simulink model "GS_Flare"  (R2022a)
settings: Solver=VariableStepAuto  StartTime=0.0  StopTime=180  RelTol=1e-3
values from neighbouring files (symbols this model uses):
  A_long = SS_lo.A([3 7 8 5 11], [3 7 8 5 11])    [glideslope_flare.m]    (also in openloop_pitchrate.m = SS_lo.A([7 8 5 11], [7 8 5 11]))
  B_long = SS_lo.A([3 7 8 5 11], [13, 14])    [glideslope_flare.m]    (also in openloop_pitchrate.m = SS_lo.A([7 8 5 11], 14))
  C_long = SS_lo.C([3 7 8 5 11], [3 7 8 5 11])    [glideslope_flare.m]    (also in openloop_pitchrate.m = SS_lo.C([7 8 5 11], [7 8 5 11]))
  D_long = SS_lo.C([3 7 8 5 11], [13, 14])    [glideslope_flare.m]    (also in openloop_pitchrate.m = SS_lo.C([7 8 5 11], 14))
  ho = 9.44    [glideslope_flare.m]
  tau = 3.15    [glideslope_flare.m]
undefined symbols (not defined in the file or in its folder): magnitude
libraries: simulink_extras x3, slpidlib x1
settings Model: Creator=gabri  LastModifiedBy=gabri

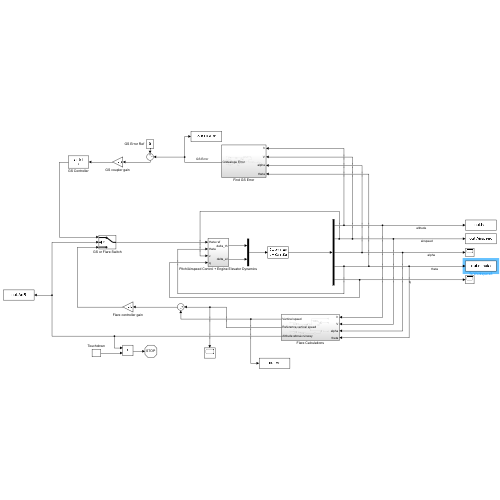
[thumbnail: Simulink's stored preview of the top-level diagram]
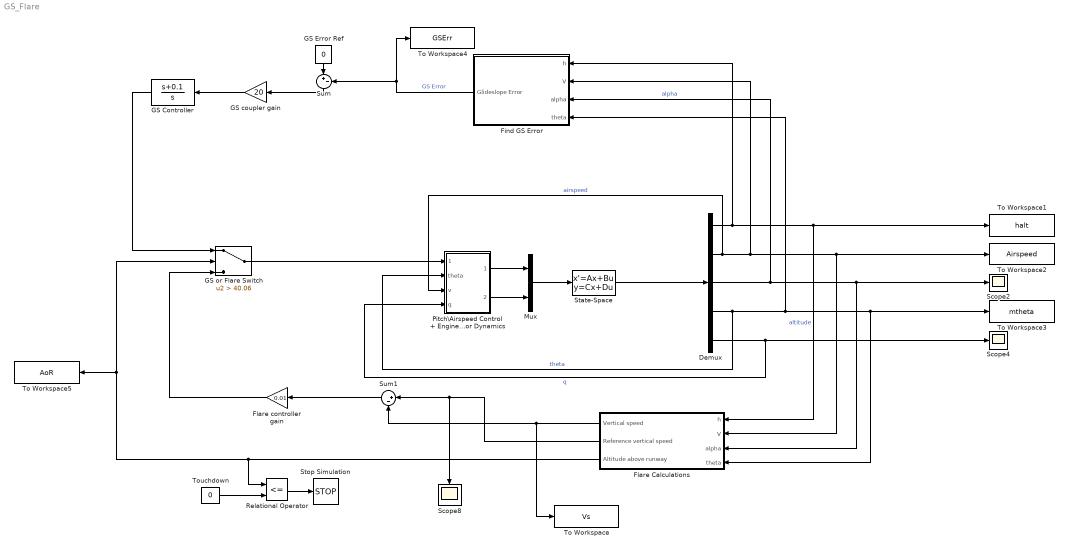
== system GS_Flare ==
  Demux : Demux  Outputs=5
  Find GS Error : Subsystem
  Flare Calculations : Subsystem
  Flare controller gain : Gain  Gain=0.01
  GS Controller : TransferFcn  Numerator=[1 0.1]  Denominator=[1 0]
  GS Error Ref : Constant  Value=0
  GS coupler gain : Gain  Gain=20
  GS or Flare Switch : Switch  Criteria=u2 > Threshold  Threshold=40.06  SaturateOnIntegerOverflow=off  InputSameDT=off
  Mux : Mux  Inputs=2
  Pitch\Airspeed Control + Engine Elevator Dynamics : Subsystem
  Relational Operator : RelationalOperator  Operator=<=  OutDataTypeStr=boolean  RndMeth=Simplest  InputSameDT=off
  Scope2 : Scope
  Scope4 : Scope
  Scope8 : Scope
  State-Space : StateSpace  A=A_long  B=B_long  C=C_long  D=D_long  InitialCondition=0
  Stop Simulation : Stop
  Sum : Sum  Inputs=|+-
  Sum1 : Sum  Inputs=|+-
  To Workspace : ToWorkspace  VariableName=Vs  SaveFormat=Timeseries  SampleTime=-1
  To Workspace1 : ToWorkspace  VariableName=halt  SaveFormat=Timeseries  SampleTime=-1
  To Workspace2 : ToWorkspace  VariableName=Airspeed  SaveFormat=Timeseries  SampleTime=-1
  To Workspace3 : ToWorkspace  VariableName=mtheta  SaveFormat=Timeseries  SampleTime=-1
  To Workspace4 : ToWorkspace  VariableName=GSErr  SaveFormat=Timeseries  SampleTime=-1
  To Workspace5 : ToWorkspace  VariableName=AoR  SaveFormat=Timeseries  SampleTime=-1
  Touchdown : Constant  Value=0
  wires:
  Demux/1 -> To Workspace1/1, Flare Calculations/1(h), Find GS Error/1(h)  "altitude"
  Demux/5 -> Pitch\Airspeed Control + Engine Elevator Dynamics/4(q), Scope4/1  "q"
  Demux/4 -> Pitch\Airspeed Control + Engine Elevator Dynamics/2(theta), To Workspace3/1, Flare Calculations/4(theta), Find GS Error/4(theta)  "theta"
  Demux/3 -> Flare Calculations/3(alpha), Scope2/1, Find GS Error/3(alpha)  "alpha"
  Demux/2 -> To Workspace2/1, Flare Calculations/2(V), Find GS Error/2(V), Pitch\Airspeed Control + Engine Elevator Dynamics/3(v)  "airspeed"
  State-Space/1 -> Demux/1
  Mux/1 -> State-Space/1
  Pitch\Airspeed Control + Engine Elevator Dynamics/2(delta_el) -> Mux/2
  Find GS Error/1(Glideslope Error) -> To Workspace4/1, Sum/2  "GS Error"
  GS Controller/1 -> GS or Flare Switch/1
  Sum/1 -> GS coupler gain/1
  GS coupler gain/1 -> GS Controller/1
  Flare Calculations/3(Altitude above runway) -> Relational Operator/1, To Workspace5/1, GS or Flare Switch/2
  Flare Calculations/2(Reference vertical speed) -> Sum1/1, Scope8/1
  Flare Calculations/1(Vertical speed) -> To Workspace/1, Sum1/2
  GS or Flare Switch/1 -> Pitch\Airspeed Control + Engine Elevator Dynamics/1(theta ref)
  GS Error Ref/1 -> Sum/1
  Relational Operator/1 -> Stop Simulation/1
  Touchdown/1 -> Relational Operator/2
  Sum1/1 -> Flare controller gain/1
  Flare controller gain/1 -> GS or Flare Switch/3
  Pitch\Airspeed Control + Engine Elevator Dynamics/1(delta_th) -> Mux/1

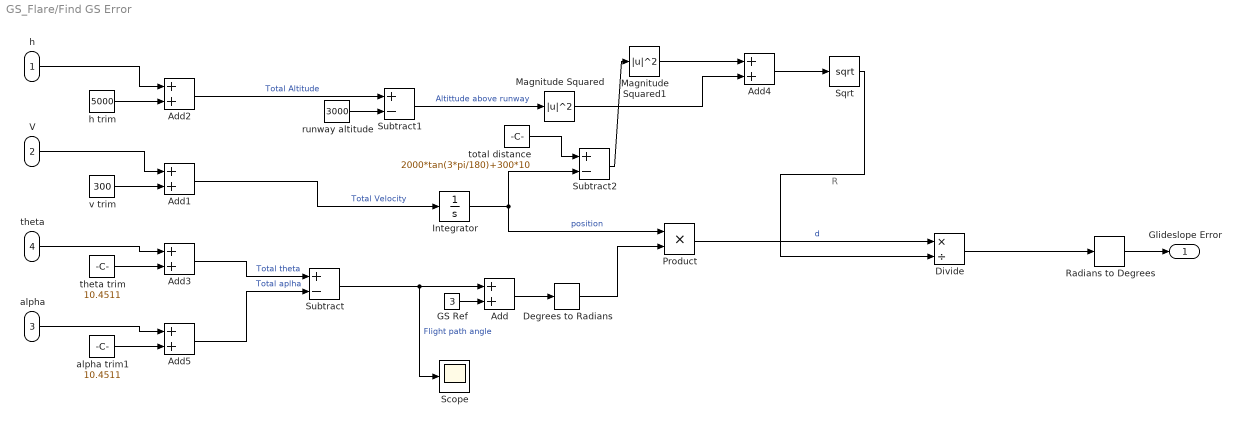
== system GS_Flare/Find GS Error ==
  note: R
  h : Inport
  V : Inport  Port=2
  alpha : Inport  Port=3
  theta : Inport  Port=4
  Add{,1..5} (6 alike) : Sum
  Degrees to Radians : simulink_extras/Transformations/Degrees to Radians
  Divide : Product  Inputs=*/
  GS Ref : Constant  Value=3
  Integrator : Integrator
  Magnitude Squared : Math  Operator=magnitude^2
  Magnitude Squared1 : Math  Operator=magnitude^2
  Product : Product
  Radians to Degrees : simulink_extras/Transformations/Radians to Degrees
  Scope : Scope
  Sqrt : Sqrt
  Subtract : Sum  Inputs=+-
  Subtract1 : Sum  Inputs=+-
  Subtract2 : Sum  Inputs=+-
  alpha trim1 : Constant  Value=10.4511
  h trim : Constant  Value=5000
  runway altitude : Constant  Value=3000
  theta trim : Constant  Value=10.4511
  total distance : Constant  Value=2000*tan(3*pi/180)+300*10
  v trim : Constant  Value=300
  Glideslope Error : Outport
  wires:
  h trim/1 -> Add2/2
  Add1/1 -> Integrator/1  "Total Velocity"
  theta/1 -> Add3/1
  V/1 -> Add1/1
  alpha trim1/1 -> Add5/2
  Product/1 -> Divide/1  "d"
  v trim/1 -> Add1/2
  Add2/1 -> Subtract1/1  "Total Altitude"
  h/1 -> Add2/1
  Radians to Degrees/1 -> Glideslope Error/1
  Subtract/1 -> Scope/1, Add/1  "Flight path angle"
  Add3/1 -> Subtract/1  "Total theta"
  Add/1 -> Degrees to Radians/1
  Degrees to Radians/1 -> Product/2
  Divide/1 -> Radians to Degrees/1
  alpha/1 -> Add5/1
  theta trim/1 -> Add3/2
  GS Ref/1 -> Add/2
  Add5/1 -> Subtract/2  "Total aplha"
  Subtract1/1 -> Magnitude Squared/1  "Altittude above runway"
  Magnitude Squared1/1 -> Add4/1
  Add4/1 -> Sqrt/1
  runway altitude/1 -> Subtract1/2
  Magnitude Squared/1 -> Add4/2
  Sqrt/1 -> Divide/2
  Integrator/1 -> Product/1, Subtract2/2  "position"
  Subtract2/1 -> Magnitude Squared1/1
  total distance/1 -> Subtract2/1

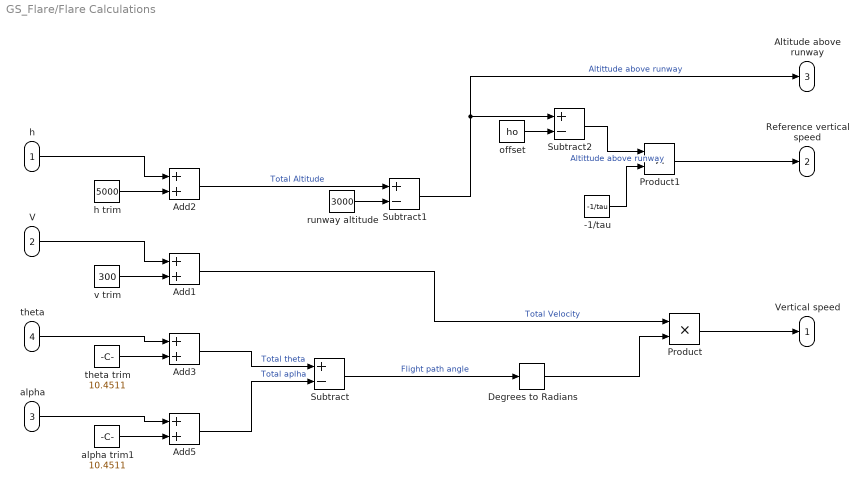
== system GS_Flare/Flare Calculations ==
  h : Inport
  V : Inport  Port=2
  alpha : Inport  Port=3
  theta : Inport  Port=4
  -1/tau : Constant  Value=-1/tau
  Add{1..3,5} (4 alike) : Sum
  Degrees to Radians : simulink_extras/Transformations/Degrees to Radians
  Product : Product
  Product1 : Product
  Subtract : Sum  Inputs=+-
  Subtract1 : Sum  Inputs=+-
  Subtract2 : Sum  Inputs=+-
  alpha trim1 : Constant  Value=10.4511
  h trim : Constant  Value=5000
  offset : Constant  Value=ho
  runway altitude : Constant  Value=3000
  theta trim : Constant  Value=10.4511
  v trim : Constant  Value=300
  Vertical speed : Outport
  Reference vertical speed : Outport  Port=2
  Altitude above runway : Outport  Port=3
  wires:
  alpha trim1/1 -> Add5/2
  -1/tau/1 -> Product1/2
  Degrees to Radians/1 -> Product/2
  Product1/1 -> Reference vertical speed/1
  theta/1 -> Add3/1
  runway altitude/1 -> Subtract1/2
  Add5/1 -> Subtract/2  "Total aplha"
  h trim/1 -> Add2/2
  alpha/1 -> Add5/1
  Subtract1/1 -> Subtract2/1, Altitude above runway/1  "Altittude above runway"
  v trim/1 -> Add1/2
  theta trim/1 -> Add3/2
  V/1 -> Add1/1
  h/1 -> Add2/1
  Add3/1 -> Subtract/1  "Total theta"
  Add2/1 -> Subtract1/1  "Total Altitude"
  Product/1 -> Vertical speed/1
  Subtract/1 -> Degrees to Radians/1  "Flight path angle"
  Add1/1 -> Product/1  "Total Velocity"
  Subtract2/1 -> Product1/1  "Altittude above runway"
  offset/1 -> Subtract2/2

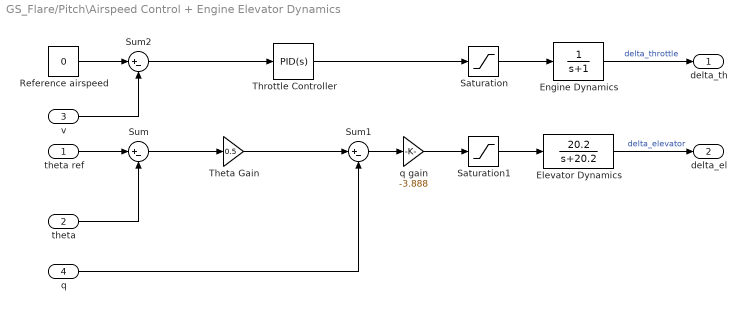
== system GS_Flare/Pitch\Airspeed Control + Engine Elevator Dynamics ==
  theta ref : Inport
  theta : Inport  Port=2
  v : Inport  Port=3
  q : Inport  Port=4
  Elevator Dynamics : TransferFcn  Numerator=[20.2]  Denominator=[1 20.2]
  Engine Dynamics : TransferFcn  Denominator=[1 1]
  Reference airspeed : Constant  Value=0
  Saturation : Saturate  UpperLimit=19000-2826.8165  LowerLimit=1000-2826.8165
  Saturation1 : Saturate  UpperLimit=25+4.1891  LowerLimit=-25+4.1891
  Sum : Sum  Inputs=|+-
  Sum1 : Sum  Inputs=|+-
  Sum2 : Sum  Inputs=|+-
  Theta Gain : Gain  Gain=0.5
  Throttle Controller : slpidlib/PID Controller  Controller=PID  Form=Parallel  TimeDomain=Continuous-time  UseExternalTs=off  SampleTime=-1  IntegratorMethod=Forward Euler  FilterMethod=Forward Euler  ControllerParametersSource=internal  P=5000  I=20  UseKiTs=off  D=100  N=100  UseFilter=on  TunerSelectOption=Transfer Function Based (PID Tuner App)  InitialConditionSource=internal  InitialConditionForIntegrator=0  InitialConditionForFilter=0  DifferentiatorICPrevScaledInput=0  ExternalReset=none  TrackingMode=off  Kt=1  LimitOutput=off  SatLimitsSource=internal  UpperSaturationLimit=inf  LowerSaturationLimit=-inf  LinearizeAsGain=on  AntiWindupMode=none  Kb=1  POutMin=[]  POutMax=[]  IOutMin=[]  IOutMax=[]  DOutMin=[]  DOutMax=[]  NOutMin=[]  NOutMax=[]  SumOutMin=[]  SumOutMax=[]  SaturationOutMin=[]  SaturationOutMax=[]  PParamMin=[]  PParamMax=[]  IParamMin=[]  IParamMax=[]  DParamMin=[]  DParamMax=[]  NParamMin=[]  NParamMax=[]  KbParamMin=[]  KbParamMax=[]  KtParamMin=[]  KtParamMax=[]  KbOutMin=[]  KbOutMax=[]  KtOutMin=[]  KtOutMax=[]  IntegratorOutMin=[]  IntegratorOutMax=[]  FilterOutMin=[]  FilterOutMax=[]  SumI1OutMin=[]  SumI1OutMax=[]  SumI2OutMin=[]  SumI2OutMax=[]  SumI3OutMin=[]  SumI3OutMax=[]  SumI4OutMin=[]  SumI4OutMax=[]  SumDOutMin=[]  SumDOutMax=[]  DifferentiatorOutMin=[]  DifferentiatorOutMax=[]  FilterDiffOutCoefMin=[]  FilterDiffOutCoefMax=[]  ReciprocalOutMin=[]  ReciprocalOutMax=[]  SumDenOutMin=[]  SumDenOutMax=[]  SumNumOutMin=[]  SumNumOutMax=[]  DivideOutMin=[]  DivideOutMax=[]  UdiffTsProdOutMin=[]  UdiffTsProdOutMax=[]  NTsProdOutMin=[]  NTsProdOutMax=[]  UintegralTsProdOutMin=[]  UintegralTsProdOutMax=[]  UngainTsProdOutMin=[]  UngainTsProdOutMax=[]  IntegratorContinuousStateAttributes=''  IntegratorStateMustResolveToSignalObject=off  IntegratorRTWStateStorageClass=Auto  FilterContinuousStateAttributes=''  FilterStateMustResolveToSignalObject=off  FilterRTWStateStorageClass=Auto  ParallelPVariant=InternalParameters  IdealPVariant=Disabled  IVariant=InternalParameters  DVariant=InternalParameters  IntegratorVariant=Continuous  SatVariant=Disabled  AWVariant=Passthrough  PCopyVariant=Disabled  TRVariant=Disabled  FdbkBlocksVariant=Forward  IdealPFdbkVariant=Disabled  SatFdbkVariant=Disabled  DerivativeFilterVariant=ContFilter  NVariant=InternalParameters  NCopyVariant=Disabled  FilterICVariant=InternalICsFilter  IntegratorICVariant=InternalICs  ExternalResetVariant=Disabled  TRSumVariant=Passthrough  SumFdbkVariant=Disabled  SumVariant=Sum_PID  TsampFilterVariant=InternalTs  TsampNgainVariant=Passthrough  TsampIntegralVariant=Passthrough  ExternalSaturationOutDataTypeStr=Inherit: Same as second input  aMode=0
  q gain : Gain  Gain=-3.888
  delta_th : Outport
  delta_el : Outport  Port=2
  wires:
  Elevator Dynamics/1 -> delta_el/1  "delta_elevator"
  Engine Dynamics/1 -> delta_th/1  "delta_throttle"
  theta ref/1 -> Sum/1
  Sum/1 -> Theta Gain/1
  Theta Gain/1 -> Sum1/1
  theta/1 -> Sum/2
  q/1 -> Sum1/2
  Sum1/1 -> q gain/1
  v/1 -> Sum2/2
  Sum2/1 -> Throttle Controller/1
  Reference airspeed/1 -> Sum2/1
  Throttle Controller/1 -> Saturation/1
  Saturation/1 -> Engine Dynamics/1
  q gain/1 -> Saturation1/1
  Saturation1/1 -> Elevator Dynamics/1
